simulink model "RegenModelV2"  (R2015b)
settings: Solver=ode4  StartTime=0.0  StopTime=inf  FixedStep=0.001  RelTol=1e-3
libraries: dsparch4 x1, simulink x1, dspsrcs4 x1
settings Model: Creator=Sven-VDR  LastModifiedBy=Sven-VDR
settings HardwareCC: ProdWordSize=32  ProdHWDeviceType=Specified

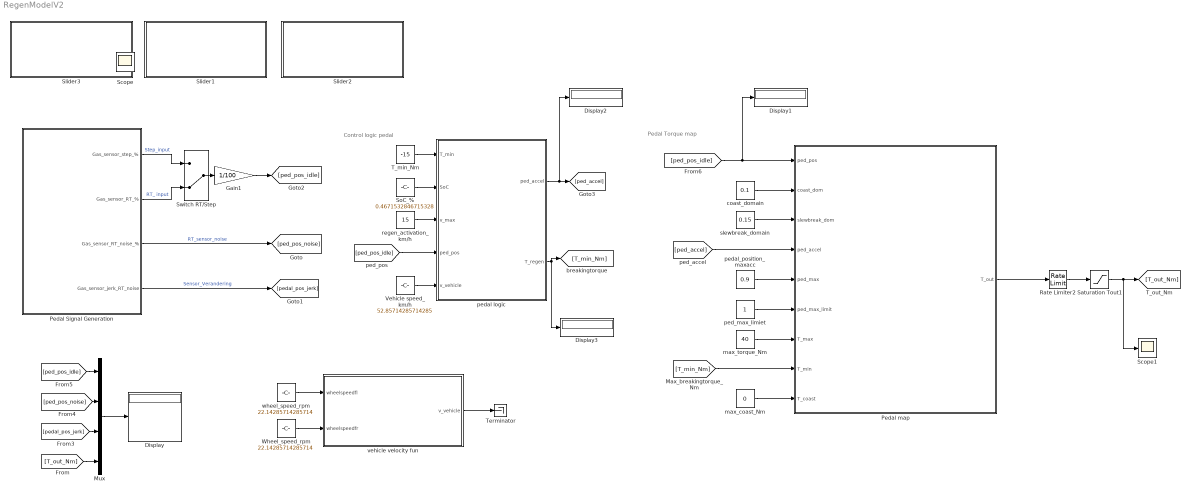
== system RegenModelV2 ==
  note: Pedal Torque map
  note: Control logic pedal
  Display{,1..3} (4 alike) : Display
  Gain1 : Gain  Gain=1/100
  Mux : Mux
  Pedal Signal Generation : Subsystem
  Pedal map : MATLAB Function  TreatAsAtomicUnit=on
  Rate Limiter2 : RateLimiter  RisingSlewLimit=20  FallingSlewLimit=-20  SampleTimeMode=inherited
  Saturation Tout1 : Saturate  UpperLimit=40  LowerLimit=-40
  Scope1 : Scope
  Slider1 : Subsystem  DialogController=hmiCreateDDGDialog  IsWebBlock=on  mask(MWDashboardBlock){webBlockId=622605c7-9e9c-405e-9f88-0fb0ede40235, webBlockType=slider, ShowInLibBrowser=on, ShowInitialText=on, HMISrcModelName=RegenModelV2}
      mask prompts: webBlockId "WebBlock Id"; webBlockType "WebBlock Type"; HMISrcModelName "Source Model"
      mask Help: helpview([docroot '/mapfiles/simulink.map'], 'hmi_slider')
      mask Display:
      | if strcmp(get_param(bdroot(gcb),'BlockDiagramType'), 'library')
      |     image([(matlabroot) '/toolbox/simulink/hmi/icons/Slider.png']);
      | end
  Slider2 : Subsystem  DialogController=hmiCreateDDGDialog  IsWebBlock=on  mask(MWDashboardBlock){webBlockId=739854d9-afda-4be6-9323-75c3d0771d11, webBlockType=slider, ShowInLibBrowser=on, ShowInitialText=on, HMISrcModelName=RegenModelV2}
      mask prompts: webBlockId "WebBlock Id"; webBlockType "WebBlock Type"; HMISrcModelName "Source Model"
      mask Help: helpview([docroot '/mapfiles/simulink.map'], 'hmi_slider')
      mask Display:
      | if strcmp(get_param(bdroot(gcb),'BlockDiagramType'), 'library')
      |     image([(matlabroot) '/toolbox/simulink/hmi/icons/Slider.png']);
      | end
  Slider3 : Subsystem  DialogController=hmiCreateDDGDialog  IsWebBlock=on  mask(MWDashboardBlock){webBlockId=5551fdec-935f-45f4-9b27-5097300807e3, webBlockType=slider, ShowInLibBrowser=on, ShowInitialText=on, HMISrcModelName=RegenModelV2}
      mask prompts: webBlockId "WebBlock Id"; webBlockType "WebBlock Type"; HMISrcModelName "Source Model"
      mask Help: helpview([docroot '/mapfiles/simulink.map'], 'hmi_slider')
      mask Display:
      | if strcmp(get_param(bdroot(gcb),'BlockDiagramType'), 'library')
      |     image([(matlabroot) '/toolbox/simulink/hmi/icons/Slider.png']);
      | end
  SoC_% : Constant  Value=0.4671532846715328
  Switch RT/Step : ManualSwitch  CurrentSetting=0
  T_min_Nm : Constant  Value=-15
  Terminator : Terminator
  Vehicle speed_km/h : Constant  Value=52.85714285714285
  Wheel_speed_rpm : Constant  Value=22.14285714285714
  coast_domain : Constant  Value=0.1
  max_coast_Nm : Constant  Value=0
  max_torque_Nm : Constant  Value=40
  ped_max_limiet : Constant
  pedal logic : Stateflow chart  TreatAsAtomicUnit=on
  pedal_position_maxacc : Constant  Value=0.9
  regen_activation_km/h : Constant  Value=15
  slewbreak_domain : Constant  Value=0.15
  vehicle velocity fun : MATLAB Function  TreatAsAtomicUnit=on
  wheel_speed_rpm : Constant  Value=22.14285714285714
  Scope : Scope
  wires:
  Switch RT/Step/1 -> Gain1/1
  Pedal Signal Generation/4(Gas_sensor_jerk_RT_noise) -> [pedal_pos_jerk]  "Sensor_Verandering"
  [pedal_pos_jerk] -> Mux/3
  [ped_pos_noise] -> Mux/2
  [ped_pos_idle] -> Mux/1
  Mux/1 -> Display/1
  Pedal Signal Generation/1(Gas_sensor_step_%) -> Switch RT/Step/1  "Step_input"
  Pedal Signal Generation/2(Gas_sensor_RT_%) -> Switch RT/Step/2  "RT_ input"
  Pedal Signal Generation/3(Gas_sensor_RT_noise_%) -> [ped_pos_noise]  "RT_sensor_noise"
  Pedal map/1(T_out) -> Rate Limiter2/1
  Rate Limiter2/1 -> Saturation Tout1/1
  coast_domain/1 -> Pedal map/2(coast_dom)
  slewbreak_domain/1 -> Pedal map/3(slewbreak_dom)
  pedal logic/1(ped_accel) -> Display2/1, [ped_accel]
  [ped_accel] -> Pedal map/4(ped_accel)
  SoC_%/1 -> pedal logic/2(SoC)
  Vehicle speed_km/h/1 -> pedal logic/5(v_vehicle)
  [ped_pos_idle] -> pedal logic/4(ped_pos)
  T_min_Nm/1 -> pedal logic/1(T_min)
  pedal_position_maxacc/1 -> Pedal map/5(ped_max)
  ped_max_limiet/1 -> Pedal map/6(ped_max_limit)
  pedal logic/2(T_regen) -> Display3/1, [T_min_Nm]
  [T_min_Nm] -> Pedal map/8(T_min)
  max_torque_Nm/1 -> Pedal map/7(T_max)
  max_coast_Nm/1 -> Pedal map/9(T_coast)
  regen_activation_km/h/1 -> pedal logic/3(v_max)
  vehicle velocity fun/1(v_vehicle) -> Terminator/1
  wheel_speed_rpm/1 -> vehicle velocity fun/1(wheelspeedfl)
  Wheel_speed_rpm/1 -> vehicle velocity fun/2(wheelspeedfr)
  Gain1/1 -> [ped_pos_idle]
  Saturation Tout1/1 -> Scope1/1, [T_out_Nm]
  [T_out_Nm] -> Mux/4
  [ped_pos_idle] -> Pedal map/1(ped_pos), Display1/1

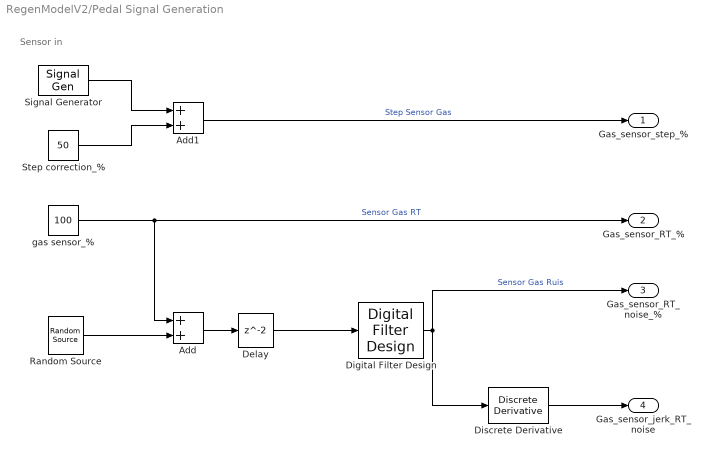
== system RegenModelV2/Pedal Signal Generation ==
  note: Sensor in
  Add : Sum
  Add1 : Sum
  Delay : Delay  SampleTime=0.001
  Digital Filter Design : dsparch4/Digital Filter Design  mwdsp_browser_bugfix_var=off
  Discrete Derivative : simulink/Discrete/Discrete Derivative  gainval=1.0  ICPrevScaledInput=0.0  InputProcessing=Inherited  OutMin=[]  OutMax=[]  OutDataType=fixdt(1, 16)  OutScaling=2^-10  DoSatur=off
  Random Source : dspsrcs4/Random Source  SrcType=Uniform  NormMethod=Ziggurat  CltLength=12  MinVal=-1  MaxVal=1  MeanVal=0  VarVal=1  RepMode=Not repeatable  rawSeed=1  IsInherit=off  SampMode=Discrete  SampTime=0.001  SampFrame=1  DataType=Double  OutComplex=Real  OutputFrames=on
  Signal Generator : SignalGenerator  WaveForm=square  Amplitude=50  Frequency=0.25
  Step correction_% : Constant  Value=50
  "gas sensor_% " : Constant  Value=100
  Gas_sensor_step_% : Outport
  Gas_sensor_RT_% : Outport  Port=2
  Gas_sensor_RT_noise_% : Outport  Port=3
  Gas_sensor_jerk_RT_noise : Outport  Port=4
  wires:
  "gas sensor_% "/1 -> Gas_sensor_RT_%/1, Add/1  "Sensor Gas RT"
  Signal Generator/1 -> Add1/1
  Add1/1 -> Gas_sensor_step_%/1  "Step Sensor Gas"
  Random Source/1 -> Add/2
  Step correction_%/1 -> Add1/2
  Add/1 -> Delay/1
  Digital Filter Design/1 -> Gas_sensor_RT_noise_%/1, Discrete Derivative/1  "Sensor Gas Ruis"
  Discrete Derivative/1 -> Gas_sensor_jerk_RT_noise/1
  Delay/1 -> Digital Filter Design/1

== system RegenModelV2/Slider1 ==

== system RegenModelV2/Slider2 ==

== system RegenModelV2/Slider3 ==

== matlab function RegenModelV2/Pedal map ==
  data: ped_pos input; coast_dom input; T_out output; slewbreak_dom input; ped_accel input; ped_max input; ped_max_limit input; T_max input; T_min input; T_coast input
function T_out = Pedalmap_eq(ped_pos,coast_dom,slewbreak_dom,ped_accel,ped_max,ped_max_limit,T_max,T_min,T_coast)
%%Accelerator pedal mapping:

ped_regen=ped_accel-coast_dom; %pedal postion - start regen - variable in function of velocity
ped_zero=ped_regen-slewbreak_dom; %pedal postion - start max regen - variable in function of velocity

slewrate_acc=(T_max-T_coast)/(ped_max-ped_accel); %slewrate acceleration region
slewrate_regen=(T_min-T_coast)/(ped_zero-ped_regen);%slewrate regen region

% acceleration pedal map eq.
T_out=T_min*(heavi(ped_pos,0)-heavi(ped_pos,ped_zero)) + (slewrate_regen*(ped_pos-ped_regen)+T_coast)*(heavi(ped_pos,ped_zero)-heavi(ped_pos,ped_regen))+T_coast*(heavi(ped_pos,ped_regen)-heavi(ped_pos,ped_accel))+(slewrate_acc*(ped_pos-ped_accel)+T_coast)*(heavi(ped_pos,ped_accel)-heavi(ped_pos,ped_max))+T_max*(heavi(ped_pos,ped_max-heavi(ped_pos,ped_max_limit)));

== matlab function RegenModelV2/vehicle velocity fun ==
  data: wheelspeedfl input; v_vehicle output; wheelspeedfr input
function v_vehicle = vehicle_velocity(wheelspeedfl,wheelspeedfr)
%% vehicle speed estimation
r=0.0254;

v_vehicle= (wheelspeedfl+wheelspeedfr)/2 *r;

== stateflow chart RegenModelV2/pedal logic ==
  state Driving
    state Disable_regen %SoC is to high.
      entry:
      ped_accel=0.45;
      T_regen=0;
    state Activate_regen
      entry:
      ped_accel=0.45;
      T0= -5; %Regentorque at v_max [Nm]
      during:
      % velocity dependant braking torque
      if v_vehicle<15
      T_regen=T_min/15
      elseif v_vehicle<50
      T_regen=T_min
      else
      T_regen=(T_min-T0)/(50-100)*(v_vehicle-100)+T0
      end
    (default) -> Disable_regen %SoC is to high.
    Disable_regen %SoC is to high. -> Activate_regen : [SoC<0.95]
    Activate_regen -> Disable_regen %SoC is to high. : [SoC>0.95]
  state Standstill
    entry:
    T_regen=0;
    ped_accel=0.1; %
    during:
    %velocity dependent coasting until v_max
    if ped_pos>0.1
    ped_accel=min(ped_pos* (v_vehicle/v_max),0.45); %Offset of 0.1
    end
    exit:
    ped_accel=0.45;
  (default) -> Standstill
  Driving -> Standstill : [v_vehicle<=3]
  Standstill -> Driving : [v_vehicle >v_max&&ped_pos>0.45]
  data: T_min input; SoC input; v_max input; ped_pos input; v_vehicle input; ped_accel output; T_regen output; T0 local
